simulink model "equalizer"  (Simulink 9.1)
settings: Solver=ode45  StartTime=0.0  StopTime=240  RelTol=1e-3  EnableMultiTasking=on
libraries: dsparch4 x8, dspmathops x8, dspvision x1, dspobslib x1
settings Model: Creator=Liza  LastModifiedBy=shami
settings DataIOCC: LimitDataPoints=on  SignalLoggingSaveFormat=ModelDataLogs
settings OptimizationCC: ExpressionDepthLimit=2147483647
settings DebuggingCC: SolverPrmCheckMsg=warning  FcnCallInpInsideContextMsg=warning  StateNameClashWarn=warning
settings GRTTargetCC: GeneratePreprocessorConditionals=Disable all

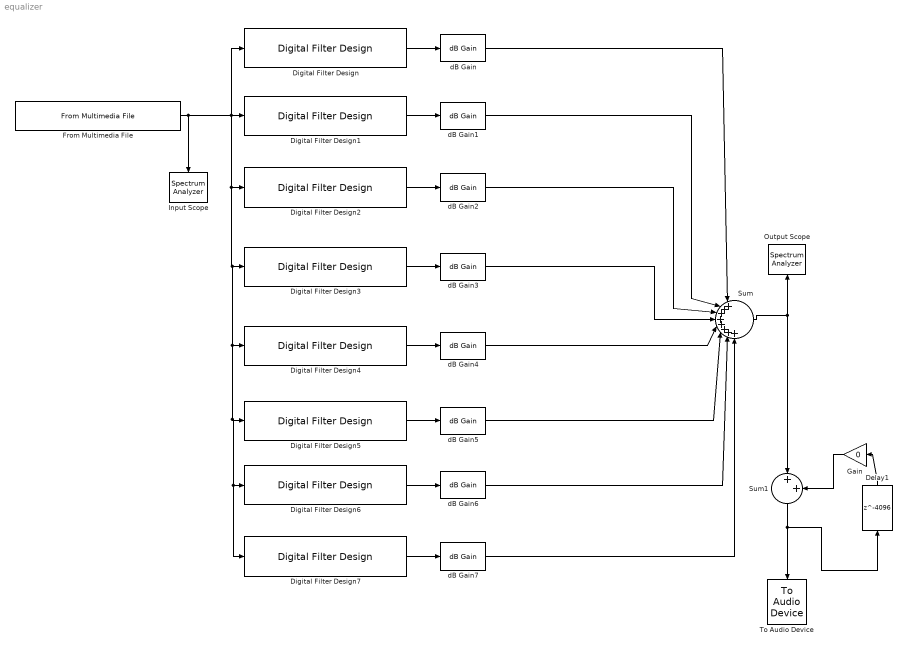
== system equalizer ==
  Delay1 : Delay  DelayLength=4096  InputProcessing=Columns as channels (frame based)
  Digital Filter Design{,1..7} (8 alike) : dsparch4/Digital Filter Design  mwdsp_browser_bugfix_var=off
  From Multimedia File : dspvision/From Multimedia File  inputFilename=C:\Users\shami\OneDrive\МГТУ\5 Семестр\ЦОС\ДЗ ЦОС\white noise.mp3  loop=on  numPlays=inf  outputStreams=Audio only  videoDataType=single  audioDataType=double  inheritSampleTime=on  userDefinedSampleTime=1/30  noAudioOutput=off  isIntensityVideo=off  fourcc=RGB  colorVideoFormat=Separate color signals  outputEOF=off  dataOrg=Column-major  audioFrameSize=1024  computeAudioFrameSize=off  outSamplingMode=Frame based
      settings: SourceProductBaseCode=VP
  Gain : Gain  Gain=0
  Input Scope : SpectrumAnalyzer
  Output Scope : SpectrumAnalyzer
  Sum : Sum  Inputs=|++++++++
  Sum1 : Sum  Inputs=|++
  To Audio Device : dspobslib/To Audio Device  deviceName=Default  inheritSampleRate=on  sampleRate=44100  deviceDatatype=Determine from input data type  autoBufferSize=on  bufferSize=4096  queueDuration=1.0  defaultOutputChannelMapping=on  outputChannelMapping=1:2  outputNumUnderrunSamples=off
      settings: SourceProductName=DSP System Toolbox  SourceProductBaseCode=DS
  dB Gain{,1..7} (8 alike) : dspmathops/dB Gain  dB=0  intype=Amplitude
      settings: SourceProductName=DSP System Toolbox  SourceProductBaseCode=DS
  wires:
  Digital Filter Design/1 -> dB Gain/1
  Digital Filter Design1/1 -> dB Gain1/1
  Digital Filter Design2/1 -> dB Gain2/1
  Digital Filter Design3/1 -> dB Gain3/1
  Digital Filter Design4/1 -> dB Gain4/1
  Digital Filter Design5/1 -> dB Gain5/1
  Sum/1 -> Output Scope/1, Sum1/1
  dB Gain/1 -> Sum/1
  dB Gain1/1 -> Sum/2
  dB Gain2/1 -> Sum/3
  dB Gain3/1 -> Sum/4
  dB Gain4/1 -> Sum/5
  dB Gain5/1 -> Sum/6
  From Multimedia File/1 -> Digital Filter Design1/1, Digital Filter Design/1, Digital Filter Design7/1, Digital Filter Design6/1, Digital Filter Design5/1, Digital Filter Design4/1, Digital Filter Design3/1, Digital Filter Design2/1, Input Scope/1
  Sum1/1 -> Delay1/1, To Audio Device/1
  Gain/1 -> Sum1/2
  Delay1/1 -> Gain/1
  Digital Filter Design6/1 -> dB Gain6/1
  Digital Filter Design7/1 -> dB Gain7/1
  dB Gain6/1 -> Sum/7
  dB Gain7/1 -> Sum/8
